simulink model "hw_mobile_robot_trajectory_control"  (R2020b)
settings: Solver=ode1  StartTime=0.0  StopTime=60  FixedStep=0.01  RelTol=1e-3  EnableMultiTasking=on
libraries: arduinolib x4, pid_lib x2, simulink x2, dspsigops x1
settings Model: SILPILModeSetting=veronly  ExtModeTrigDuration=2  Creator=ONLY-GOD  LastModifiedBy=ONLY-GOD
settings OptimizationCC: EnhancedBackFolding=on  PassReuseOutputArgsAs=Individual arguments  ZeroExternalMemoryAtStartup=off  ZeroInternalMemoryAtStartup=off  MaxStackSize=64  OptimizeBlockOrder=speed  DifferentSizesBufferReuse=on  OptimizationCustomize=off  EfficientTunableParamExpr=on
settings DebuggingCC: ParameterTunabilityLossMsg=error
settings HardwareCC: ProdBitPerPointer=32  ProdBitPerSizeT=32  ProdBitPerPtrDiffT=32  ProdLargestAtomicInteger=Long  ProdLargestAtomicFloat=Double  ProdWordSize=32  ProdHWDeviceType=ARM Compatible->ARM Cortex
settings SFSimCC: MATLABDynamicMemAlloc=off
settings RTWCC: Description=Embedded Coder  SystemTargetFile=ert.tlc  HardwareBoard=Arduino Due  TemplateMakefile=ert_default_tmf  Toolchain=Arduino ARM  BuildConfiguration=Faster Runs
settings CodeAppCC: ForceParamTrailComments=on  IgnoreCustomStorageClasses=off  OperatorAnnotations=on  SimulinkDataObjDesc=on  SFDataObjDesc=on  InsertBlockDesc=on
settings ERTTargetCC: SupportContinuousTime=on  SupportVariableSizeSignals=on  ExtModeTransport=3  ExtModeStaticAllocSize=24576  ExtModeMexFile=ext_xcp  ExtModeIntrfLevel=Level2 - Open

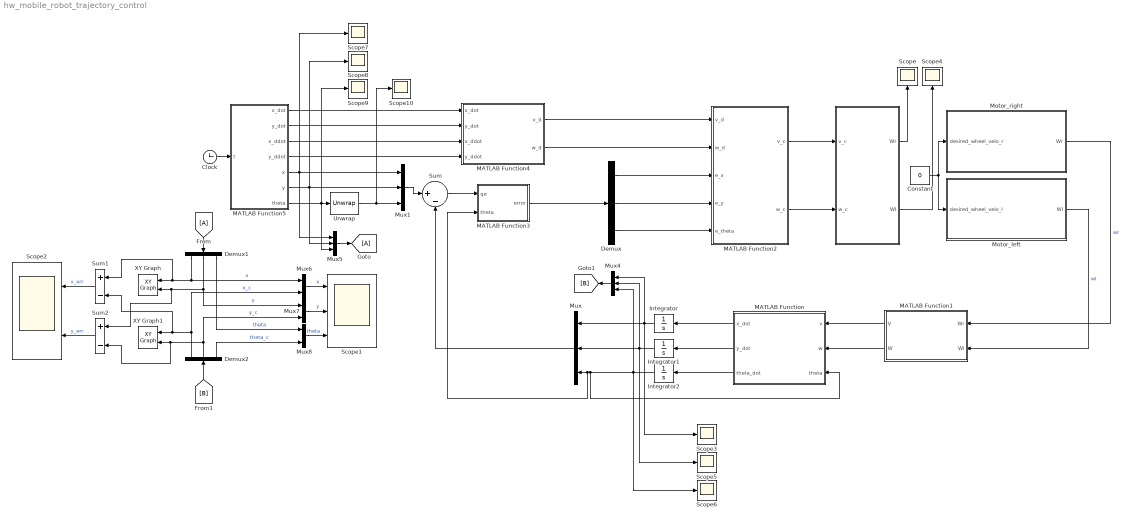
== system hw_mobile_robot_trajectory_control ==
  " " : MATLAB Function  TreatAsAtomicUnit=on
  Clock : Clock
  Constant : Constant  Value=0
  Demux : Demux  Outputs=3
  Demux1 : Demux  Outputs=3
  Demux2 : Demux  Outputs=3
  Integrator : Integrator
  Integrator1 : Integrator
  Integrator2 : Integrator
  MATLAB Function : MATLAB Function  TreatAsAtomicUnit=on
  MATLAB Function1 : MATLAB Function  TreatAsAtomicUnit=on
  MATLAB Function2 : MATLAB Function  TreatAsAtomicUnit=on
  MATLAB Function3 : MATLAB Function  TreatAsAtomicUnit=on
  MATLAB Function4 : MATLAB Function  TreatAsAtomicUnit=on
  MATLAB Function5 : MATLAB Function  TreatAsAtomicUnit=on
  Motor_left : Subsystem
  Motor_right : Subsystem
  Mux{,1,4..5} (4 alike) : Mux  Inputs=3
  Mux6 : Mux  Inputs=2
  Mux7 : Mux  Inputs=2
  Mux8 : Mux  Inputs=2
  Scope{,3..10} (9 alike) : Scope
  Scope1 : Scope  NumInputPorts=3
  Scope2 : Scope  NumInputPorts=2
  Sum : Sum  Inputs=|+-
  Sum1 : Sum  Inputs=+-
  Sum2 : Sum  Inputs=+-
  Unwrap : dspsigops/Unwrap  tol=pi  InputProcessing=Columns as channels (frame based)  running=off
  XY Graph : simulink/Sinks/XY Graph  xmin=-6  xmax=6  ymin=-6  ymax=6  st=-1
  XY Graph1 : simulink/Sinks/XY Graph  xmin=-6  xmax=6  ymin=-6  ymax=6  st=-1
  wires:
  Demux/1 -> MATLAB Function2/3(e_x)
  Demux/2 -> MATLAB Function2/4(e_y)
  Demux/3 -> MATLAB Function2/5(e_theta)
  Sum/1 -> MATLAB Function3/1(qe)
  MATLAB Function3/1(error) -> Demux/1
  MATLAB Function4/1(v_d) -> MATLAB Function2/1(v_d)
  MATLAB Function4/2(w_d) -> MATLAB Function2/2(w_d)
  MATLAB Function2/1(v_c) -> " "/1(v_c)
  MATLAB Function2/2(w_c) -> " "/2(w_c)
  Motor_right/1(Wr) -> MATLAB Function1/1(Wr)  "wr"
  Motor_left/1(Wl) -> MATLAB Function1/2(Wl)  "wl"
  MATLAB Function1/1(V) -> MATLAB Function/1(v)
  MATLAB Function1/2(W) -> MATLAB Function/2(w)
  MATLAB Function/3(theta_dot) -> Integrator2/1
  MATLAB Function/1(x_dot) -> Integrator/1
  MATLAB Function/2(y_dot) -> Integrator1/1
  Integrator2/1 -> Scope6/1, Mux4/3, Mux/3, MATLAB Function3/2(theta), MATLAB Function/3(theta)
  Integrator1/1 -> Mux/2, Scope5/1, Mux4/2
  Mux/1 -> Sum/2
  MATLAB Function5/1(x_dot) -> MATLAB Function4/1(x_dot)
  MATLAB Function5/2(y_dot) -> MATLAB Function4/2(y_dot)
  MATLAB Function5/3(x_ddot) -> MATLAB Function4/3(x_ddot)
  MATLAB Function5/4(y_ddot) -> MATLAB Function4/4(y_ddot)
  Clock/1 -> MATLAB Function5/1(t)
  MATLAB Function5/5(x) -> Mux1/1, Mux5/1, Scope7/1
  MATLAB Function5/6(y) -> Mux1/2, Mux5/2, Scope8/1
  MATLAB Function5/7(theta) -> Scope9/1, Mux5/3, Unwrap/1
  Mux1/1 -> Sum/1
  Mux5/1 -> [A]
  Mux4/1 -> [B]
  [A] -> Demux1/1
  [B] -> Demux2/1
  Demux1/1 -> Sum1/1, XY Graph/1, Mux6/1  "x"
  Demux2/1 -> XY Graph1/1, Sum1/2, Mux6/2  "x_c"
  Demux1/2 -> Sum2/1, XY Graph/2, Mux7/1  "y"
  Demux2/2 -> Sum2/2, XY Graph1/2, Mux7/2  "y_c"
  Demux2/3 -> Mux8/2  "theta_c"
  Mux6/1 -> Scope1/1  "x"
  Mux7/1 -> Scope1/2  "y"
  Mux8/1 -> Scope1/3  "theta"
  Demux1/3 -> Mux8/1  "theta"
  Sum1/1 -> Scope2/1  "x_err"
  Sum2/1 -> Scope2/2  "y_err"
  Constant/1 -> Motor_left/1(desired_wheel_velo_l), Motor_right/1(desired_wheel_velo_r)
  Integrator/1 -> Mux/1, Scope3/1, Mux4/1
  Unwrap/1 -> Scope10/1, Mux1/3
  " "/1(Wr) -> Scope/1
  " "/2(Wl) -> Scope4/1

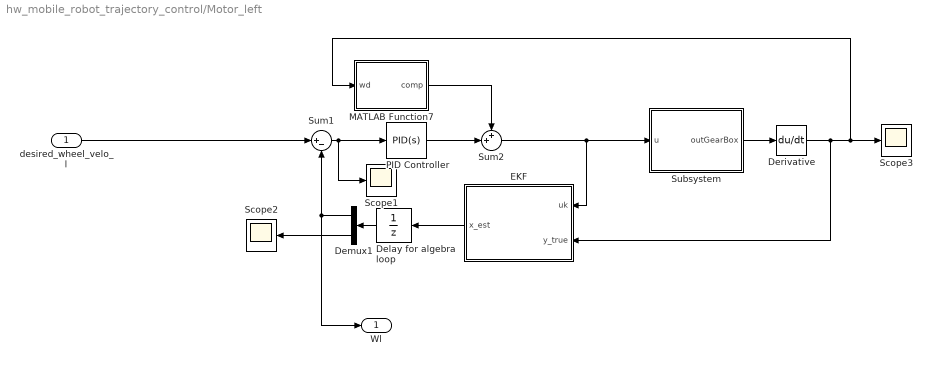
== system hw_mobile_robot_trajectory_control/Motor_left ==
  desired_wheel_velo_l : Inport
  Delay for algebra loop : UnitDelay  SampleTime=-1  HasFrameUpgradeWarning=on
  Demux1 : Demux  Outputs=[1,3]
  Derivative : Derivative
  EKF : MATLAB Function  TreatAsAtomicUnit=on
  MATLAB Function7 : MATLAB Function  TreatAsAtomicUnit=on
  PID Controller : pid_lib/PID Controller  Controller=PID  Form=Parallel  TimeDomain=Continuous-time  UseExternalTs=off  SampleTime=-1  IntegratorMethod=Forward Euler  FilterMethod=Forward Euler  ControllerParametersSource=internal  P=3*(27.65*(-1+2*1.5-2*sqrt(1.5*(1.5-1)))/17.35)  I=3*(27.65*(-1+2*1.5-2*sqrt(1.5*(1.5-1)))/17.35)* 1.5*27.65  D=0  UseFilter=on  N=100  TunerSelectOption=Transfer Function Based (PID Tuner App)  InitialConditionSource=internal  InitialConditionForIntegrator=0  InitialConditionForFilter=0  DifferentiatorICPrevScaledInput=0  ExternalReset=none  TrackingMode=off  Kt=1  LimitOutput=off  SatLimitsSource=internal  UpperSaturationLimit=inf  LowerSaturationLimit=-inf  LinearizeAsGain=on  AntiWindupMode=none  Kb=1  POutMin=[]  POutMax=[]  IOutMin=[]  IOutMax=[]  DOutMin=[]  DOutMax=[]  NOutMin=[]  NOutMax=[]  SumOutMin=[]  SumOutMax=[]  SaturationOutMin=[]  SaturationOutMax=[]  PParamMin=[]  PParamMax=[]  IParamMin=[]  IParamMax=[]  DParamMin=[]  DParamMax=[]  NParamMin=[]  NParamMax=[]  KbParamMin=[]  KbParamMax=[]  KtParamMin=[]  KtParamMax=[]  KbOutMin=[]  KbOutMax=[]  KtOutMin=[]  KtOutMax=[]  IntegratorOutMin=[]  IntegratorOutMax=[]  FilterOutMin=[]  FilterOutMax=[]  SumI1OutMin=[]  SumI1OutMax=[]  SumI2OutMin=[]  SumI2OutMax=[]  SumI3OutMin=[]  SumI3OutMax=[]  SumI4OutMin=[]  SumI4OutMax=[]  SumDOutMin=[]  SumDOutMax=[]  DifferentiatorOutMin=[]  DifferentiatorOutMax=[]  FilterDiffOutCoefMin=[]  FilterDiffOutCoefMax=[]  ReciprocalOutMin=[]  ReciprocalOutMax=[]  SumDenOutMin=[]  SumDenOutMax=[]  SumNumOutMin=[]  SumNumOutMax=[]  DivideOutMin=[]  DivideOutMax=[]  UdiffTsProdOutMin=[]  UdiffTsProdOutMax=[]  NTsProdOutMin=[]  NTsProdOutMax=[]  UintegralTsProdOutMin=[]  UintegralTsProdOutMax=[]  UngainTsProdOutMin=[]  UngainTsProdOutMax=[]  IntegratorContinuousStateAttributes=''  IntegratorStateMustResolveToSignalObject=off  IntegratorRTWStateStorageClass=Auto  FilterContinuousStateAttributes=''  FilterStateMustResolveToSignalObject=off  FilterRTWStateStorageClass=Auto  ParallelPVariant=InternalParameters  IdealPVariant=Disabled  IVariant=InternalParameters  DVariant=InternalParameters  IntegratorVariant=Continuous  SatVariant=Disabled  AWVariant=Passthrough  PCopyVariant=Disabled  TRVariant=Disabled  FdbkBlocksVariant=Forward  IdealPFdbkVariant=Disabled  SatFdbkVariant=Disabled  DerivativeFilterVariant=ContFilter  NVariant=InternalParameters  NCopyVariant=Disabled  FilterICVariant=InternalICsFilter  IntegratorICVariant=InternalICs  ExternalResetVariant=Disabled  TRSumVariant=Passthrough  SumFdbkVariant=Disabled  SumVariant=Sum_PID  TsampFilterVariant=InternalTs  TsampNgainVariant=Passthrough  TsampIntegralVariant=Passthrough  ExternalSaturationOutDataTypeStr=Inherit: Same as second input
  Scope1 : Scope
  Scope2 : Scope
  Scope3 : Scope
  Subsystem : Subsystem
  Sum1 : Sum  Inputs=|+-
  Sum2 : Sum  Inputs=++|
  Wl : Outport
  wires:
  Delay for algebra loop/1 -> Demux1/1
  Demux1/1 -> Sum1/2, Wl/1
  MATLAB Function7/1(comp) -> Sum2/1
  Demux1/2 -> Scope2/1
  EKF/1(x_est) -> Delay for algebra loop/1
  PID Controller/1 -> Sum2/2
  Sum1/1 -> PID Controller/1, Scope1/1
  desired_wheel_velo_l/1 -> Sum1/1
  Sum2/1 -> Subsystem/1(u), EKF/1(uk)
  Subsystem/1(outGearBox) -> Derivative/1
  Derivative/1 -> MATLAB Function7/1(wd), Scope3/1, EKF/2(y_true)

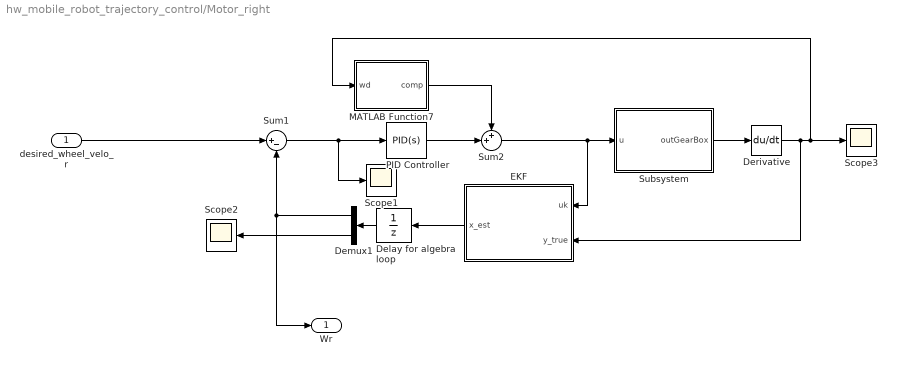
== system hw_mobile_robot_trajectory_control/Motor_right ==
  desired_wheel_velo_r : Inport
  Delay for algebra loop : UnitDelay  SampleTime=-1  HasFrameUpgradeWarning=on
  Demux1 : Demux  Outputs=[1,3]
  Derivative : Derivative
  EKF : MATLAB Function  TreatAsAtomicUnit=on
  MATLAB Function7 : MATLAB Function  TreatAsAtomicUnit=on
  PID Controller : pid_lib/PID Controller  Controller=PID  Form=Parallel  TimeDomain=Continuous-time  UseExternalTs=off  SampleTime=-1  IntegratorMethod=Forward Euler  FilterMethod=Forward Euler  ControllerParametersSource=internal  P=3*(27.65*(-1+2*1.5-2*sqrt(1.5*(1.5-1)))/17.35)  I=3*(27.65*(-1+2*1.5-2*sqrt(1.5*(1.5-1)))/17.35)* 1.5*27.65  D=0  UseFilter=on  N=100  TunerSelectOption=Transfer Function Based (PID Tuner App)  InitialConditionSource=internal  InitialConditionForIntegrator=0  InitialConditionForFilter=0  DifferentiatorICPrevScaledInput=0  ExternalReset=none  TrackingMode=off  Kt=1  LimitOutput=off  SatLimitsSource=internal  UpperSaturationLimit=inf  LowerSaturationLimit=-inf  LinearizeAsGain=on  AntiWindupMode=none  Kb=1  POutMin=[]  POutMax=[]  IOutMin=[]  IOutMax=[]  DOutMin=[]  DOutMax=[]  NOutMin=[]  NOutMax=[]  SumOutMin=[]  SumOutMax=[]  SaturationOutMin=[]  SaturationOutMax=[]  PParamMin=[]  PParamMax=[]  IParamMin=[]  IParamMax=[]  DParamMin=[]  DParamMax=[]  NParamMin=[]  NParamMax=[]  KbParamMin=[]  KbParamMax=[]  KtParamMin=[]  KtParamMax=[]  KbOutMin=[]  KbOutMax=[]  KtOutMin=[]  KtOutMax=[]  IntegratorOutMin=[]  IntegratorOutMax=[]  FilterOutMin=[]  FilterOutMax=[]  SumI1OutMin=[]  SumI1OutMax=[]  SumI2OutMin=[]  SumI2OutMax=[]  SumI3OutMin=[]  SumI3OutMax=[]  SumI4OutMin=[]  SumI4OutMax=[]  SumDOutMin=[]  SumDOutMax=[]  DifferentiatorOutMin=[]  DifferentiatorOutMax=[]  FilterDiffOutCoefMin=[]  FilterDiffOutCoefMax=[]  ReciprocalOutMin=[]  ReciprocalOutMax=[]  SumDenOutMin=[]  SumDenOutMax=[]  SumNumOutMin=[]  SumNumOutMax=[]  DivideOutMin=[]  DivideOutMax=[]  UdiffTsProdOutMin=[]  UdiffTsProdOutMax=[]  NTsProdOutMin=[]  NTsProdOutMax=[]  UintegralTsProdOutMin=[]  UintegralTsProdOutMax=[]  UngainTsProdOutMin=[]  UngainTsProdOutMax=[]  IntegratorContinuousStateAttributes=''  IntegratorStateMustResolveToSignalObject=off  IntegratorRTWStateStorageClass=Auto  FilterContinuousStateAttributes=''  FilterStateMustResolveToSignalObject=off  FilterRTWStateStorageClass=Auto  ParallelPVariant=InternalParameters  IdealPVariant=Disabled  IVariant=InternalParameters  DVariant=InternalParameters  IntegratorVariant=Continuous  SatVariant=Disabled  AWVariant=Passthrough  PCopyVariant=Disabled  TRVariant=Disabled  FdbkBlocksVariant=Forward  IdealPFdbkVariant=Disabled  SatFdbkVariant=Disabled  DerivativeFilterVariant=ContFilter  NVariant=InternalParameters  NCopyVariant=Disabled  FilterICVariant=InternalICsFilter  IntegratorICVariant=InternalICs  ExternalResetVariant=Disabled  TRSumVariant=Passthrough  SumFdbkVariant=Disabled  SumVariant=Sum_PID  TsampFilterVariant=InternalTs  TsampNgainVariant=Passthrough  TsampIntegralVariant=Passthrough  ExternalSaturationOutDataTypeStr=Inherit: Same as second input
  Scope1 : Scope
  Scope2 : Scope
  Scope3 : Scope
  Subsystem : Subsystem
  Sum1 : Sum  Inputs=|+-
  Sum2 : Sum  Inputs=++|
  Wr : Outport
  wires:
  Sum2/1 -> Subsystem/1(u), EKF/1(uk)
  desired_wheel_velo_r/1 -> Sum1/1
  Sum1/1 -> Scope1/1, PID Controller/1
  PID Controller/1 -> Sum2/2
  EKF/1(x_est) -> Delay for algebra loop/1
  Demux1/2 -> Scope2/1
  MATLAB Function7/1(comp) -> Sum2/1
  Demux1/1 -> Wr/1, Sum1/2
  Delay for algebra loop/1 -> Demux1/1
  Subsystem/1(outGearBox) -> Derivative/1
  Derivative/1 -> MATLAB Function7/1(wd), Scope3/1, EKF/2(y_true)

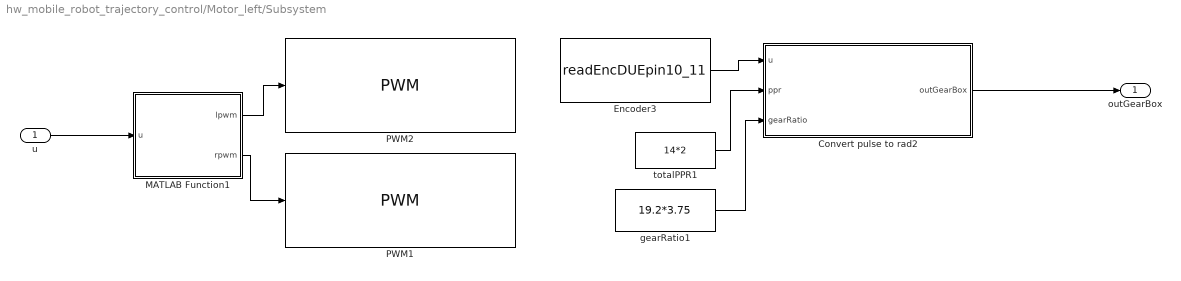
== system hw_mobile_robot_trajectory_control/Motor_left/Subsystem ==
  u : Inport
  Convert pulse to rad2 : MATLAB Function  TreatAsAtomicUnit=on
  Encoder3 : S-Function  InitFcn=try, set_param(gcb,'FunctionName','readEncDUEpin10_11'), end  FunctionName=readEncDUEpin10_11  SFunctionModules=readEncDUEpin10_11_wrapper  SFunctionDeploymentMode=off  EnableBusSupport=off  mask(S-Function Builder){}
      mask help: Simulink:masks:SFunctionBuilder_MD
      mask init:
      | val = [[.9  0.75 0.75 1 1 .9 .9 1]',[1 1 0.75 0.75 .9 .9 1 .9]'];try , sys = get_param(gcb,'SfunBuilderFcnName');if isempty(sys), sys = get_param(gcb,'FunctionName'); end,catch, sys = get_param(gcb,'FunctionName'); end
      settings: CopyFcn=set_param(gcbh,'LinkStatus','none')  PreSaveFcn=try, set_param(gcb,'FunctionName','readEncDUEpin10_11'), end  OpenFcn=sfunctionwizard(gcbh)
      mask Display: plot(val(:,1),val(:,2)),disp(sys),port_label('output',1,'countt')
  MATLAB Function1 : MATLAB Function  TreatAsAtomicUnit=on
  PWM1 : arduinolib/PWM  pinNumber=4  frequencyType=Default  desiredFrequency=490.2  achievableFrequency=490.2
  PWM2 : arduinolib/PWM  pinNumber=5  frequencyType=Default  desiredFrequency=490.2  achievableFrequency=490.2
  gearRatio1 : Constant  Value=19.2*3.75
  totalPPR1 : Constant  Value=14*2
  outGearBox : Outport
  wires:
  Encoder3/1 -> Convert pulse to rad2/1(u)
  totalPPR1/1 -> Convert pulse to rad2/2(ppr)
  gearRatio1/1 -> Convert pulse to rad2/3(gearRatio)
  Convert pulse to rad2/1(outGearBox) -> outGearBox/1
  MATLAB Function1/1(lpwm) -> PWM2/1
  MATLAB Function1/2(rpwm) -> PWM1/1
  u/1 -> MATLAB Function1/1(u)

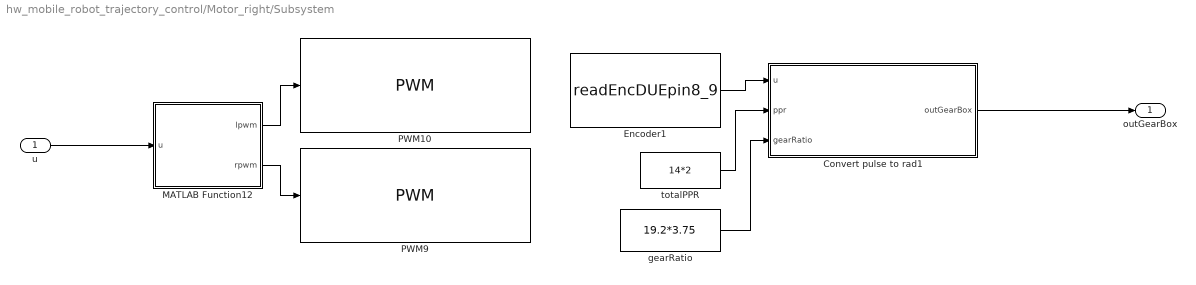
== system hw_mobile_robot_trajectory_control/Motor_right/Subsystem ==
  u : Inport
  Convert pulse to rad1 : MATLAB Function  TreatAsAtomicUnit=on
  Encoder1 : S-Function  InitFcn=try, set_param(gcb,'FunctionName','readEncDUEpin8_9'), end  FunctionName=readEncDUEpin8_9  SFunctionModules=readEncDUEpin8_9_wrapper  SFunctionDeploymentMode=off  EnableBusSupport=off  mask(S-Function Builder){}
      mask help: Simulink:masks:SFunctionBuilder_MD
      mask init: same as hw_mobile_robot_trajectory_control/Motor_left/Subsystem/Encoder3
      settings: CopyFcn=set_param(gcbh,'LinkStatus','none')  PreSaveFcn=try, set_param(gcb,'FunctionName','readEncDUEpin8_9'), end  OpenFcn=sfunctionwizard(gcbh)
      mask Display: plot(val(:,1),val(:,2)),disp(sys),port_label('output',1,'count')
  MATLAB Function12 : MATLAB Function  TreatAsAtomicUnit=on
  PWM10 : arduinolib/PWM  pinNumber=7  frequencyType=Default  desiredFrequency=490.2  achievableFrequency=490.2
  PWM9 : arduinolib/PWM  pinNumber=6  frequencyType=Default  desiredFrequency=490.2  achievableFrequency=490.2
  gearRatio : Constant  Value=19.2*3.75
  totalPPR : Constant  Value=14*2
  outGearBox : Outport
  wires:
  gearRatio/1 -> Convert pulse to rad1/3(gearRatio)
  MATLAB Function12/2(rpwm) -> PWM9/1
  MATLAB Function12/1(lpwm) -> PWM10/1
  totalPPR/1 -> Convert pulse to rad1/2(ppr)
  Encoder1/1 -> Convert pulse to rad1/1(u)
  Convert pulse to rad1/1(outGearBox) -> outGearBox/1
  u/1 -> MATLAB Function12/1(u)

== matlab function hw_mobile_robot_trajectory_control/Motor_right/Subsystem/Convert pulse to rad1 ==
  settings: updateMethod=DISCRETE
  data: u input; ppr input; gearRatio input; outGearBox output
function outGearBox = fcn(u,ppr,gearRatio)

persistent counter_num over_flag
if(isempty(counter_num)), counter_num = 0;end
if(isempty(over_flag)), over_flag = 0;end
pulse2radian = 2*pi/ppr; % 1 pulse = ?? radian

if(double(u) - counter_num > 40000), over_flag = over_flag-1;
elseif(double(u) - counter_num < -40000), over_flag = over_flag+1;
end

inGearBox = (double(u)+over_flag*(2^32 -1))*pulse2radian; 
outGearBox = inGearBox/gearRatio;
counter_num = double(u) ;

== matlab function hw_mobile_robot_trajectory_control/Motor_left/Subsystem/Convert pulse to rad2 ==
  settings: updateMethod=DISCRETE
  data: u input; ppr input; gearRatio input; outGearBox output
function outGearBox = fcn(u,ppr,gearRatio)

persistent counter_num over_flag
if(isempty(counter_num)), counter_num = 0;end
if(isempty(over_flag)), over_flag = 0;end
pulse2radian = 2*pi/ppr; % 1 pulse = ?? radian

if(double(u) - counter_num > 40000), over_flag = over_flag-1;
elseif(double(u) - counter_num < -40000), over_flag = over_flag+1;
end

inGearBox = (double(u)+over_flag*(2^32 -1))*pulse2radian; 
outGearBox = inGearBox/gearRatio;
counter_num = double(u) ;

== matlab function hw_mobile_robot_trajectory_control/Motor_right/Subsystem/MATLAB Function12 ==
  data: u input; lpwm output; rpwm output
function [lpwm,rpwm] = fcn(u)

Vmax = 22.9;
pwm = u*254/Vmax;
if pwm > 0
    lpwm = pwm;
    rpwm = 0;
elseif pwm < 0
    lpwm = 0;
    rpwm = abs(pwm);
else
    lpwm = 0;
    rpwm = 0;
end

== matlab function hw_mobile_robot_trajectory_control/Motor_left/EKF ==
  settings: updateMethod=DISCRETE
  data: uk input; y_true input; x_est output
function x_est = EKF(uk,y_true)
Ts=0.01;
persistent x_est_p P Qd_est R_est Qc_est;
if isempty(x_est_p)
    
    x_est_p=[2;13;25;1];
    P=2*eye(4);
    Qc_est=1e-5*diag([10,25,25,1]);
    Qd_est=Qc_est*Ts;
    R_est=0.02;
end
c=[1 0 0 0];D=0;Ck=c;Dk=D;
%Comput Kalman Gain and update predicted value
Wk=P*Ck'/(Ck*P*Ck'+R_est);
y_est=Ck*x_est_p+Dk*uk;
x=x_est_p+Wk.*(y_true-y_est);
%Compute prediction at next time step
x_est=x+Ts*[-x(2)*x(1)+uk*x(3)-x(4)*sign(x(1));0;0;0];
%Update error covariance matrices
P=P-Wk*Ck*P;
%Define Ak
Ak=eye(4)+Ts*[-x(2) -x(1) uk -sign(x(1));0 0 0 0;0 0 0 0;0 0 0 0]; % jacobian
P=Ak*P*Ak'+Qd_est;
x_est_p=x_est;

== matlab function hw_mobile_robot_trajectory_control/Motor_left/Subsystem/MATLAB Function1 ==
  data: u input; lpwm output; rpwm output
function [lpwm,rpwm] = fcn(u)

Vmax = 22.9;
pwm = u*254/Vmax;
if pwm > 0
    lpwm = pwm;
    rpwm = 0;
elseif pwm < 0
    lpwm = 0;
    rpwm = abs(pwm);
else
    lpwm = 0;
    rpwm = 0;
end

== matlab function hw_mobile_robot_trajectory_control/  ==
  data: v_c input; Wr output; w_c input; Wl output
function [Wr, Wl] = M_inv(v_c, w_c)
r = 0.07;      %wheel radius
b = 0.22;      %length from wheel to wheel

Wr = ((2*v_c)+(w_c*b))/(2*r);
Wl = ((2*v_c)-(w_c*b))/(2*r);

== matlab function hw_mobile_robot_trajectory_control/MATLAB Function ==
  data: v input; x_dot output; w input; y_dot output; theta_dot output; theta input
function [x_dot,y_dot,theta_dot]= kinematic(v,w,theta)
x_dot = v*cos(theta);
y_dot = v*sin(theta);
theta_dot = w;

== matlab function hw_mobile_robot_trajectory_control/MATLAB Function2 ==
  data: v_d input; v_c output; w_d input; e_x input; e_y input; e_theta input; w_c output
function [v_c,w_c] =  bckstep(v_d, w_d, e_x, e_y, e_theta)            

% control gain
k1 = 1;
k2 = 20 ;
k3 = 1 ;

v_c = k1*e_x + v_d*cos(e_theta);
w_c = w_d + k2*v_d*e_y + k3*v_d*sin(e_theta);

== matlab function hw_mobile_robot_trajectory_control/MATLAB Function3 ==
  data: qe input; error output; theta input
function error = rotation(qe,theta)

T = [cos(theta) , sin(theta) , 0 ;
    -sin(theta) , cos(theta) , 0 ;
         0      ,     0      , 1 ];
     
error = T*qe;

== matlab function hw_mobile_robot_trajectory_control/MATLAB Function4 ==
  data: x_dot input; v_d output; w_d output; y_dot input; x_ddot input; y_ddot input
function [v_d,w_d] = fcn(x_dot,y_dot,x_ddot,y_ddot)

v_d = sqrt(x_dot^2 + y_dot^2);
w_d = ((x_dot*y_ddot)-(y_dot*x_ddot))/((x_dot^2 + y_dot^2));

== matlab function hw_mobile_robot_trajectory_control/Motor_right/EKF ==
  settings: updateMethod=DISCRETE
  data: uk input; y_true input; x_est output
function x_est = EKF(uk,y_true)
Ts=0.01;
persistent x_est_p P Qd_est R_est Qc_est;
if isempty(x_est_p)
    
    x_est_p=[2;13;25;1];
    P=2*eye(4);
    Qc_est=1e-5*diag([10,25,25,1]);
    Qd_est=Qc_est*Ts;
    R_est=0.02;
end
c=[1 0 0 0];D=0;Ck=c;Dk=D;
%Comput Kalman Gain and update predicted value
Wk=P*Ck'/(Ck*P*Ck'+R_est);
y_est=Ck*x_est_p+Dk*uk;
x=x_est_p+Wk.*(y_true-y_est);
%Compute prediction at next time step
x_est=x+Ts*[-x(2)*x(1)+uk*x(3)-x(4)*sign(x(1));0;0;0];
%Update error covariance matrices
P=P-Wk*Ck*P;
%Define Ak
Ak=eye(4)+Ts*[-x(2) -x(1) uk -sign(x(1));0 0 0 0;0 0 0 0;0 0 0 0]; % jacobian
P=Ak*P*Ak'+Qd_est;
x_est_p=x_est;

== matlab function hw_mobile_robot_trajectory_control/Motor_right/MATLAB Function7 ==
  settings: updateMethod=DISCRETE
  data: wd input; comp output
function comp = fcn(wd)

b = 17.35 + rand; c = 5.63 + 0.3*rand;
comp = c/b*sign(wd);

== matlab function hw_mobile_robot_trajectory_control/Motor_left/MATLAB Function7 ==
  settings: updateMethod=DISCRETE
  data: wd input; comp output
function comp = fcn(wd)

b = 17.35 + rand; c = 5.63 + 0.3*rand;
comp = c/b*sign(wd);

== matlab function hw_mobile_robot_trajectory_control/MATLAB Function1 ==
  data: Wr input; V output; Wl input; W output
function [V,W]= fcn(Wr,Wl)
r = 0.07;      %wheel radius
b = 0.22;      %length from wheel to wheel

V = r*(Wr/2) + r*(Wl/2);
W = r*(Wr/b) - r*(Wl/b);

== matlab function hw_mobile_robot_trajectory_control/MATLAB Function5 ==
  data: x_dot output; y_dot output; x_ddot output; y_ddot output; x output; t input; y output; theta output
function [x_dot,y_dot,x_ddot,y_ddot,x,y,theta] = ref(t)

f = 0.05;
r = 4;

x = r*cos(f*t);
y = r*sin(f*t);

x_dot = -r*f*sin(f*t);
y_dot = r*f*cos(f*t);

theta = atan2(y_dot,x_dot);

x_ddot = -r*f^2*cos(f*t);
y_ddot = -r*f^2*sin(f*t);
